simulink model "power_plant_simulink"  (R2012b)
settings: Solver=ode23s  StartTime=0.0  StopTime=300  FixedStep=0.01  RelTol=1e-3
undefined symbols (not defined in the file): A, B, C, D, step1_final, step1_initial, step1_time, step2_final, step2_initial, step2_time, x0
settings Model: Creator=michal  LastModifiedBy=MatCven
settings DataIOCC: SignalLoggingSaveFormat=ModelDataLogs
settings DebuggingCC: FcnCallInpInsideContextMsg=UseLocalSettings
settings GRTTargetCC: CombineOutputUpdateFcns=off  GRTInterface=on

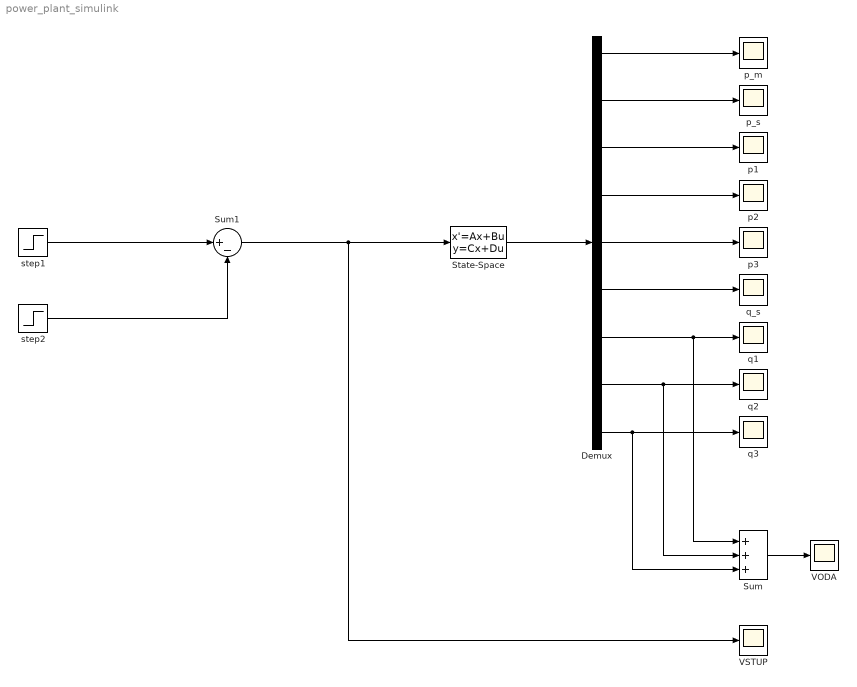
== system power_plant_simulink ==
  Demux : Demux  Outputs=9
  State-Space : StateSpace  A=A  B=B  C=C  D=D  X0=x0
  Sum : Sum  Inputs=+++
  Sum1 : Sum  Inputs=|+-
  VODA : Scope
      settings: SaveName=ScopeData6
  VSTUP : Scope
      settings: SaveName=scope_input
  p1 : Scope
      settings: SaveName=ScopeData3
  p2 : Scope
      settings: SaveName=ScopeData2
  p3 : Scope
      settings: TimeRange=300  YMin=0  YMax=5e-06
  p_m : Scope
      settings: SaveName=ScopeData5
  p_s : Scope
      settings: SaveName=ScopeData4
  q1 : Scope
      settings: SaveName=scope_prva_nadrz
  q2 : Scope
      settings: TimeRange=1000  YMin=0  YMax=0.0006000000000000001  SaveName=scope_druha_nadrz
  q3 : Scope
      settings: SaveName=scope_tretia_nadrz
  q_s : Scope
  step1 : Step  Time=step1_time  Before=step1_initial  After=step1_final  SampleTime=0
  step2 : Step  Time=step2_time  Before=step2_initial  After=step2_final  SampleTime=0
  wires:
  State-Space/1 -> Demux/1
  Demux/1 -> p_m/1
  Demux/2 -> p_s/1
  Demux/3 -> p1/1
  Demux/4 -> p2/1
  Demux/5 -> p3/1
  Demux/6 -> q_s/1
  Sum/1 -> VODA/1
  Demux/7 -> Sum/1, q1/1
  Demux/8 -> Sum/2, q2/1
  Demux/9 -> Sum/3, q3/1
  step1/1 -> Sum1/1
  Sum1/1 -> VSTUP/1, State-Space/1
  step2/1 -> Sum1/2
